simulink model "W_client_ClientServer_Model"  (R2024b)
settings: Solver=FixedStepDiscrete  StartTime=0.0  StopTime=10.0  FixedStep=0.05  RelTol=1e-3
undefined symbols (not defined in the file or in its folder): DataA, DataB, ServerService
settings Model: Tag=EP_AA_WRAPPER_SERVER  DataDictionary=Wrapper_ClientServer_Model.sldd  Creator=yatishc  LastModifiedBy=yatishc
settings OptimizationCC: DefaultParameterBehavior=Inlined  EnhancedBackFolding=on  PassReuseOutputArgsAs=Individual arguments  ZeroExternalMemoryAtStartup=off  ZeroInternalMemoryAtStartup=off  OptimizeBlockOrder=speed  DifferentSizesBufferReuse=on  OptimizationCustomize=off  EfficientTunableParamExpr=on
settings DebuggingCC: ParameterTunabilityLossMsg=error
settings SFSimCC: SimGenImportedTypeDefs=on  MATLABDynamicMemAlloc=off  SimTargetLang=C++
settings RTWCC: Description=Embedded Coder  SystemTargetFile=ert.tlc  GenCodeOnly=on  TemplateMakefile=ert_default_tmf  CustomSourceCode="#include \"ClientServer_Model_adapter.h\""  CustomInitializer=sut_initialize();  DataTypeReplacement=CDataTypesFixedWidth  TargetLang=C++
settings CodeAppCC: ForceParamTrailComments=on  IgnoreCustomStorageClasses=off  MaxIdLength=256  OperatorAnnotations=on  SimulinkDataObjDesc=on  SFDataObjDesc=on  CustomSymbolStrGlobalVar=w_$R$N$M  CustomSymbolStrType=w_$N$R$M_T  InsertBlockDesc=on
settings ERTTargetCC: TargetLangStandard=C++17 (ISO)  GenerateSampleERTMain=on  ERTCustomFileTemplate=example_file_process.tlc  MaxIdInt64=INT64_MAX  MinIdInt64=INT64_MIN  MaxIdUint64=UINT64_MAX  MaxIdInt32=INT32_MAX  MinIdInt32=INT32_MIN  MaxIdUint32=UINT32_MAX  MaxIdInt16=INT16_MAX  MinIdInt16=INT16_MIN  MaxIdUint16=UINT16_MAX  MaxIdInt8=INT8_MAX  MinIdInt8=INT8_MIN  MaxIdUint8=UINT8_MAX

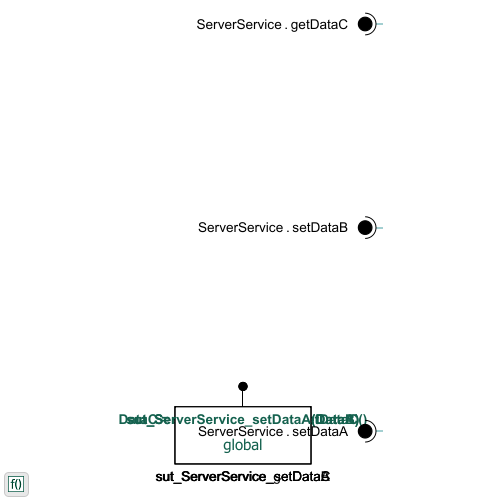
[thumbnail: Simulink's stored preview of the top-level diagram]
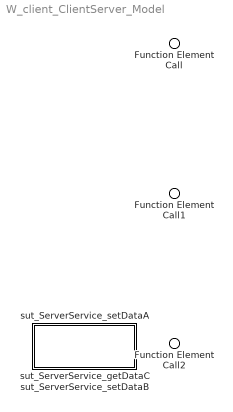
== system W_client_ClientServer_Model ==
  Function Element Call : Inport  AllowServiceAccess=on  PortName=ServerService  Element=getDataC
  Function Element Call1 : Inport  AllowServiceAccess=on  PortName=ServerService  Element=setDataB
  Function Element Call2 : Inport  AllowServiceAccess=on  PortName=ServerService  Element=setDataA
  sut_ServerService_getDataC : Subsystem  TreatAsAtomicUnit=on
  sut_ServerService_setDataA : Subsystem  TreatAsAtomicUnit=on
  sut_ServerService_setDataB : Subsystem  TreatAsAtomicUnit=on

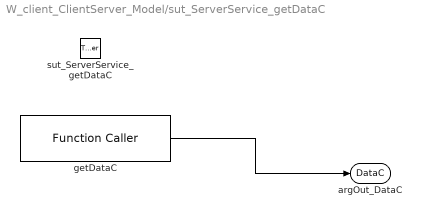
== system W_client_ClientServer_Model/sut_ServerService_getDataC ==
  sut_ServerService_getDataC : TriggerPort  TriggerType=function-call  IsSimulinkFunction=on  FunctionName=sut_ServerService_getDataC  VariantControl=(inherit)
  getDataC : FunctionCaller  FunctionPrototype=DataC = ServerService.getDataC()  OutputArgumentSpecifications=double(0)
  argOut_DataC : ArgOut  ArgumentName=DataC
  wires:
  getDataC/1 -> argOut_DataC/1

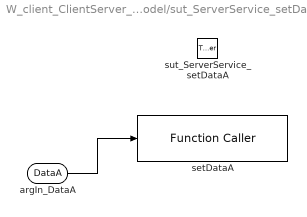
== system W_client_ClientServer_Model/sut_ServerService_setDataA ==
  sut_ServerService_setDataA : TriggerPort  TriggerType=function-call  IsSimulinkFunction=on  FunctionName=sut_ServerService_setDataA  VariantControl=(inherit)
  setDataA : FunctionCaller  FunctionPrototype=ServerService.setDataA(DataA)  InputArgumentSpecifications=double(0)
  argIn_DataA : ArgIn  ArgumentName=DataA
  wires:
  argIn_DataA/1 -> setDataA/1

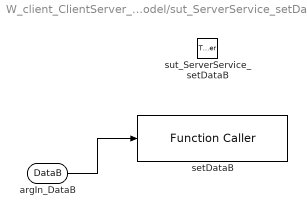
== system W_client_ClientServer_Model/sut_ServerService_setDataB ==
  sut_ServerService_setDataB : TriggerPort  TriggerType=function-call  IsSimulinkFunction=on  FunctionName=sut_ServerService_setDataB  VariantControl=(inherit)
  setDataB : FunctionCaller  FunctionPrototype=ServerService.setDataB(DataB)  InputArgumentSpecifications=double(0)
  argIn_DataB : ArgIn  ArgumentName=DataB
  wires:
  argIn_DataB/1 -> setDataB/1
